simulink model "PLL_single"  (R2022a)
settings: Solver=VariableStepAuto  StartTime=0.0  StopTime=1.2  RelTol=1e-3
InitFcn:
  | w0 = 377; Kp=180; Ki=3200;
settings Model: Creator=PSCAD_FAN  LastModifiedBy=PSCAD_FAN

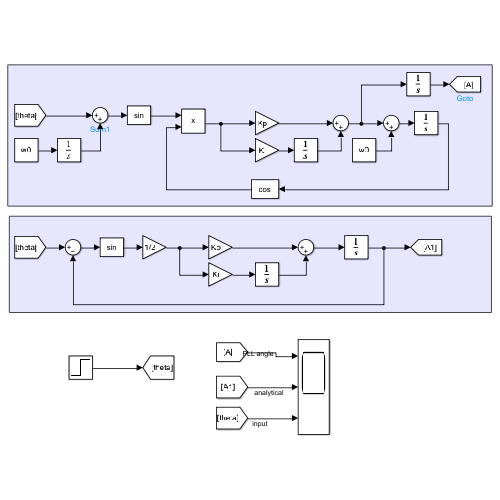
[thumbnail: Simulink's stored preview of the top-level diagram]
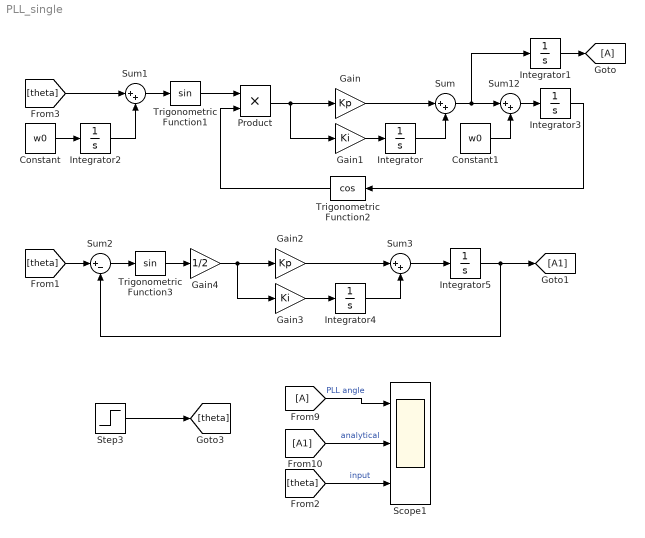
== system PLL_single ==
  Constant : Constant  Value=w0
  Constant1 : Constant  Value=w0
  From9 : From
  Gain : Gain  Gain=Kp
  Gain1 : Gain  Gain=Ki
  Gain2 : Gain  Gain=Kp
  Gain3 : Gain  Gain=Ki
  Gain4 : Gain  Gain=1/2
  Goto : Goto
  Integrator{,1..5} (6 alike) : Integrator
  Product : Product
  Scope1 : Scope  NumInputPorts=3
  Step3 : Step  After=0.5  SampleTime=0
  Sum{,1,3,12} (4 alike) : Sum  Inputs=|++
  Sum2 : Sum  Inputs=|+-
  Trigonometric Function1 : Trigonometry
  Trigonometric Function2 : Trigonometry  Operator=cos
  Trigonometric Function3 : Trigonometry
  wires:
  Integrator2/1 -> Sum1/2
  Trigonometric Function2/1 -> Product/2
  Integrator3/1 -> Trigonometric Function2/1
  Constant1/1 -> Sum12/2
  Sum12/1 -> Integrator3/1
  Trigonometric Function1/1 -> Product/1
  Integrator1/1 -> Goto/1
  Sum1/1 -> Trigonometric Function1/1
  Sum/1 -> Sum12/1, Integrator1/1
  Integrator/1 -> Sum/2
  Product/1 -> Gain1/1, Gain/1
  Gain/1 -> Sum/1
  Gain1/1 -> Integrator/1
  [theta] -> Sum1/1
  Constant/1 -> Integrator2/1
  [theta] -> Sum2/1
  Sum2/1 -> Trigonometric Function3/1
  Integrator5/1 -> [A1], Sum2/2
  Sum3/1 -> Integrator5/1
  Integrator4/1 -> Sum3/2
  Gain2/1 -> Sum3/1
  Gain3/1 -> Integrator4/1
  Trigonometric Function3/1 -> Gain4/1
  From9/1 -> Scope1/1  "PLL angle"
  [A1] -> Scope1/2  "analytical"
  Step3/1 -> [theta]
  [theta] -> Scope1/3  "input"
  Gain4/1 -> Gain3/1, Gain2/1
